simulink model "cosmic_ray_system_top"  (R2019a)
settings: Solver=VariableStepAuto  StartTime=0.0  StopTime=10.0  RelTol=1e-3
libraries: xbsIndex_r4 x3434, casper_library_misc x148, xps_library x3, casper_library_delays x1
(part 10 of 27)

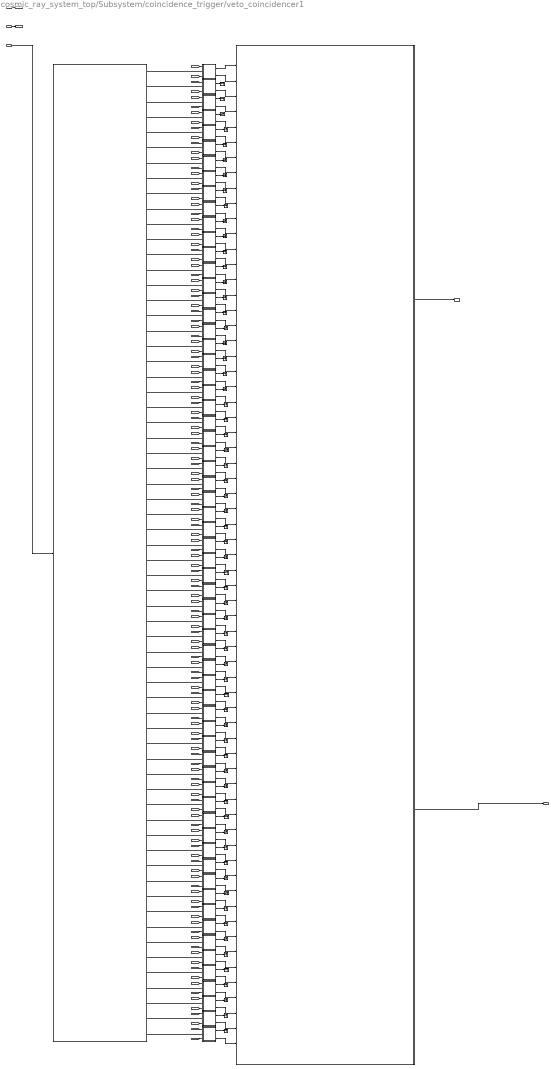
== system cosmic_ray_system_top/Subsystem/coincidence_trigger/veto_coincidencer1 ==
  window_length : Inport
  data_bus_in : Inport  Port=2
  sync_in : Inport  Port=3
  Terminator{,1..62} (63 alike) : Terminator
  adder_tree : Subsystem  AncestorBlock=casper_library_misc/adder_tree  mask(adder_tree){n_inputs=64, csp_latency=1, adder_imp=Fabric, first_stage_hdl=on, floating_point=off, dvalid_en=off, float_type=single, frac_width=0, exp_width=0}
      mask prompts: n_inputs "Number of Inputs"; csp_latency "Add Latency"; adder_imp "Adder implementation"; first_stage_hdl "Use behavioural HDL for first stage of adders"; floating_point "floating point"; float_type "float type"; frac_width "fraction length"; exp_width "exponent length"
      mask help:
      | Sums all inputs using a tree of adds and delays.
      |
      | Number of inputs: The number of inputs to the block to be summed
      | Add latency: The number of clock cycles to perform one addition (affects timing)..
      | Adder implementation: choice of fabric or DSP48E core, or behavioral HDL
      | Use behavioural HDL for first stage of adders: Causes the first stage of adders to be absorbed into DSP blocks if multipliers precede them (Virtex 5). Overrides Adder implementation
      mask init: same as cosmic_ray_system_top/Subsystem/coincidence_trigger/veto_coincidencer/adder_tree
      settings: AttributesFormatString=latency 6
      mask Help: eval('xlWeb(''http://casper.berkeley.edu/wiki/Adder_tree'')')
      mask TypeOptions adder_imp: Behavioral | Fabric | DSP48
      mask Callback floating_point:
      | onoff = get_param(gcb, 'floating_point');
      | if strcmp(onoff,'on')
      |     enable_fixpt = 'off'
      |     set_param_state(gcb, 'float_type', 'on')
      | 
      |     f_type = get_param(gcb, 'float_type')
      |     if strcmp(f_type,'custom')
      |         set_param_state(gcb, 'exp_width', 'on')
      |         set_param_state(gcb, 'frac_width', 'on')
      |     else
      |         set_param_state(gcb, 'exp_width', 'off')
      |         set_param_state(gcb, 'frac_width', 'off')
      |     end
      | 
      | 
      | else
      |     enable_fixpt = 'on'
      |     set_param_state(gcb, 'float_type', 'off')
      |     set_param_state(gcb, 'exp_width', 'off')
      |     set_param_state(gcb, 'frac_width', 'off')
      | end
      mask TypeOptions float_type: single | custom
      mask Callback float_type:
      | f_type = get_param(gcb, 'float_type')
      | if strcmp(f_type,'custom')
      |     set_param_state(gcb, 'exp_width', 'on')
      |     set_param_state(gcb, 'frac_width', 'on')
      | else
      |     set_param_state(gcb, 'exp_width', 'off')
      |     set_param_state(gcb, 'frac_width', 'off')
      | end
  bus_expand : Subsystem  AncestorBlock=casper_library_flow_control/bus_expand  mask(bus_expand){mode=divisions of equal size, outputNum=64, outputWidth=1, outputBinaryPt=0, outputArithmeticType=0, show_format=off, outputToWorkspace=off, variablePrefix=out, outputToModelAsWell=on}
      mask prompts: outputNum "Number of outputs:"; outputWidth "Output width:"; outputBinaryPt "Output binary point position:"; outputArithmeticType "Output arithmetic type (ufix=0, fix=1, bool=2):"; show_format "Print format string?"; outputToWorkspace "Output to workspace?"; variablePrefix "Variable name prefix:"; outputToModelAsWell "Output to model as well?"
      mask help:
      | Expands a 'bus' made using a bus_create or Xilinx
      | concat block.
      | The input will be divided into the specified number
      | of outputs with the specified arithmetic types.
      | Divisions are made from most significant bit.
      mask init: same as cosmic_ray_system_top/Subsystem/buffer_and_packetizer/bus_expand
      settings: AttributesFormatString=64 outputs
      mask TypeOptions mode: divisions of equal size | divisions of arbitrary size
      mask Callback mode: bus_expand_callback();
      mask Callback outputWidth: bus_expand_callback();
      mask Callback outputToWorkspace: bus_expand_callback();
  custom_pulse_extend_with_sync1 : Subsystem
  custom_pulse_extend_with_sync10 : Subsystem
  custom_pulse_extend_with_sync11 : Subsystem
  custom_pulse_extend_with_sync12 : Subsystem
  custom_pulse_extend_with_sync13 : Subsystem
  custom_pulse_extend_with_sync14 : Subsystem
  custom_pulse_extend_with_sync15 : Subsystem
  custom_pulse_extend_with_sync16 : Subsystem
  custom_pulse_extend_with_sync17 : Subsystem
  custom_pulse_extend_with_sync18 : Subsystem
  custom_pulse_extend_with_sync19 : Subsystem
  custom_pulse_extend_with_sync2 : Subsystem
  custom_pulse_extend_with_sync20 : Subsystem
  custom_pulse_extend_with_sync21 : Subsystem
  custom_pulse_extend_with_sync22 : Subsystem
  custom_pulse_extend_with_sync23 : Subsystem
  custom_pulse_extend_with_sync24 : Subsystem
  custom_pulse_extend_with_sync25 : Subsystem
  custom_pulse_extend_with_sync26 : Subsystem
  custom_pulse_extend_with_sync27 : Subsystem
  custom_pulse_extend_with_sync28 : Subsystem
  custom_pulse_extend_with_sync29 : Subsystem
  custom_pulse_extend_with_sync3 : Subsystem
  custom_pulse_extend_with_sync30 : Subsystem
  custom_pulse_extend_with_sync31 : Subsystem
  custom_pulse_extend_with_sync32 : Subsystem
  custom_pulse_extend_with_sync33 : Subsystem
  custom_pulse_extend_with_sync34 : Subsystem
  custom_pulse_extend_with_sync35 : Subsystem
  custom_pulse_extend_with_sync36 : Subsystem
  custom_pulse_extend_with_sync37 : Subsystem
  custom_pulse_extend_with_sync38 : Subsystem
  custom_pulse_extend_with_sync39 : Subsystem
  custom_pulse_extend_with_sync4 : Subsystem
  custom_pulse_extend_with_sync40 : Subsystem
  custom_pulse_extend_with_sync41 : Subsystem
  custom_pulse_extend_with_sync42 : Subsystem
  custom_pulse_extend_with_sync43 : Subsystem
  custom_pulse_extend_with_sync44 : Subsystem
  custom_pulse_extend_with_sync45 : Subsystem
  custom_pulse_extend_with_sync46 : Subsystem
  custom_pulse_extend_with_sync47 : Subsystem
  custom_pulse_extend_with_sync48 : Subsystem
  custom_pulse_extend_with_sync49 : Subsystem
  custom_pulse_extend_with_sync5 : Subsystem
  custom_pulse_extend_with_sync50 : Subsystem
  custom_pulse_extend_with_sync51 : Subsystem
  custom_pulse_extend_with_sync52 : Subsystem
  custom_pulse_extend_with_sync53 : Subsystem
  custom_pulse_extend_with_sync54 : Subsystem
  custom_pulse_extend_with_sync55 : Subsystem
  custom_pulse_extend_with_sync56 : Subsystem
  custom_pulse_extend_with_sync57 : Subsystem
  custom_pulse_extend_with_sync58 : Subsystem
  custom_pulse_extend_with_sync59 : Subsystem
  custom_pulse_extend_with_sync6 : Subsystem
  custom_pulse_extend_with_sync60 : Subsystem
  custom_pulse_extend_with_sync61 : Subsystem
  custom_pulse_extend_with_sync62 : Subsystem
  custom_pulse_extend_with_sync63 : Subsystem
  custom_pulse_extend_with_sync64 : Subsystem
  custom_pulse_extend_with_sync7 : Subsystem
  custom_pulse_extend_with_sync8 : Subsystem
  custom_pulse_extend_with_sync9 : Subsystem
  sync_out : Outport
  "out " : Outport  Port=2
  wires:
  custom_pulse_extend_with_sync63/2("out ") -> adder_tree/65(din64)
  custom_pulse_extend_with_sync64/2("out ") -> adder_tree/64(din63)
  custom_pulse_extend_with_sync61/2("out ") -> adder_tree/63(din62)
  custom_pulse_extend_with_sync62/2("out ") -> adder_tree/62(din61)
  custom_pulse_extend_with_sync44/2("out ") -> adder_tree/61(din60)
  custom_pulse_extend_with_sync45/2("out ") -> adder_tree/60(din59)
  custom_pulse_extend_with_sync41/2("out ") -> adder_tree/59(din58)
  custom_pulse_extend_with_sync43/2("out ") -> adder_tree/58(din57)
  custom_pulse_extend_with_sync39/2("out ") -> adder_tree/57(din56)
  custom_pulse_extend_with_sync40/2("out ") -> adder_tree/56(din55)
  custom_pulse_extend_with_sync54/2("out ") -> adder_tree/55(din54)
  custom_pulse_extend_with_sync51/2("out ") -> adder_tree/54(din53)
  custom_pulse_extend_with_sync52/2("out ") -> adder_tree/53(din52)
  custom_pulse_extend_with_sync49/2("out ") -> adder_tree/52(din51)
  custom_pulse_extend_with_sync50/2("out ") -> adder_tree/51(din50)
  custom_pulse_extend_with_sync47/2("out ") -> adder_tree/50(din49)
  custom_pulse_extend_with_sync48/2("out ") -> adder_tree/49(din48)
  custom_pulse_extend_with_sync38/2("out ") -> adder_tree/48(din47)
  custom_pulse_extend_with_sync46/2("out ") -> adder_tree/47(din46)
  custom_pulse_extend_with_sync36/2("out ") -> adder_tree/46(din45)
  custom_pulse_extend_with_sync37/2("out ") -> adder_tree/45(din44)
  custom_pulse_extend_with_sync34/2("out ") -> adder_tree/44(din43)
  custom_pulse_extend_with_sync35/2("out ") -> adder_tree/43(din42)
  custom_pulse_extend_with_sync32/2("out ") -> adder_tree/42(din41)
  custom_pulse_extend_with_sync33/2("out ") -> adder_tree/41(din40)
  custom_pulse_extend_with_sync60/2("out ") -> adder_tree/40(din39)
  custom_pulse_extend_with_sync58/2("out ") -> adder_tree/39(din38)
  custom_pulse_extend_with_sync59/2("out ") -> adder_tree/38(din37)
  custom_pulse_extend_with_sync56/2("out ") -> adder_tree/37(din36)
  custom_pulse_extend_with_sync57/2("out ") -> adder_tree/36(din35)
  custom_pulse_extend_with_sync53/2("out ") -> adder_tree/35(din34)
  custom_pulse_extend_with_sync55/2("out ") -> adder_tree/34(din33)
  custom_pulse_extend_with_sync31/2("out ") -> adder_tree/33(din32)
  custom_pulse_extend_with_sync42/2("out ") -> adder_tree/32(din31)
  custom_pulse_extend_with_sync21/2("out ") -> adder_tree/31(din30)
  custom_pulse_extend_with_sync22/2("out ") -> adder_tree/30(din29)
  custom_pulse_extend_with_sync19/2("out ") -> adder_tree/29(din28)
  custom_pulse_extend_with_sync20/2("out ") -> adder_tree/28(din27)
  custom_pulse_extend_with_sync17/2("out ") -> adder_tree/27(din26)
  custom_pulse_extend_with_sync18/2("out ") -> adder_tree/26(din25)
  custom_pulse_extend_with_sync30/2("out ") -> adder_tree/25(din24)
  custom_pulse_extend_with_sync28/2("out ") -> adder_tree/24(din23)
  custom_pulse_extend_with_sync29/2("out ") -> adder_tree/23(din22)
  custom_pulse_extend_with_sync26/2("out ") -> adder_tree/22(din21)
  custom_pulse_extend_with_sync27/2("out ") -> adder_tree/21(din20)
  custom_pulse_extend_with_sync24/2("out ") -> adder_tree/20(din19)
  custom_pulse_extend_with_sync25/2("out ") -> adder_tree/19(din18)
  custom_pulse_extend_with_sync16/2("out ") -> adder_tree/18(din17)
  custom_pulse_extend_with_sync23/2("out ") -> adder_tree/17(din16)
  custom_pulse_extend_with_sync14/2("out ") -> adder_tree/16(din15)
  custom_pulse_extend_with_sync15/2("out ") -> adder_tree/15(din14)
  custom_pulse_extend_with_sync12/2("out ") -> adder_tree/14(din13)
  custom_pulse_extend_with_sync13/2("out ") -> adder_tree/13(din12)
  custom_pulse_extend_with_sync10/2("out ") -> adder_tree/12(din11)
  custom_pulse_extend_with_sync11/2("out ") -> adder_tree/11(din10)
  custom_pulse_extend_with_sync9/2("out ") -> adder_tree/10(din9)
  custom_pulse_extend_with_sync7/2("out ") -> adder_tree/9(din8)
  custom_pulse_extend_with_sync8/2("out ") -> adder_tree/8(din7)
  custom_pulse_extend_with_sync5/2("out ") -> adder_tree/7(din6)
  custom_pulse_extend_with_sync6/2("out ") -> adder_tree/6(din5)
  custom_pulse_extend_with_sync3/2("out ") -> adder_tree/5(din4)
  custom_pulse_extend_with_sync4/2("out ") -> adder_tree/4(din3)
  custom_pulse_extend_with_sync1/2("out ") -> adder_tree/3(din2)
  custom_pulse_extend_with_sync2/2("out ") -> adder_tree/2(din1)
  custom_pulse_extend_with_sync44/1(sync_out) -> Terminator61/1
  custom_pulse_extend_with_sync62/1(sync_out) -> Terminator62/1
  custom_pulse_extend_with_sync61/1(sync_out) -> Terminator58/1
  custom_pulse_extend_with_sync64/1(sync_out) -> Terminator59/1
  custom_pulse_extend_with_sync63/1(sync_out) -> Terminator60/1
  custom_pulse_extend_with_sync45/1(sync_out) -> Terminator55/1
  custom_pulse_extend_with_sync41/1(sync_out) -> Terminator54/1
  custom_pulse_extend_with_sync43/1(sync_out) -> Terminator53/1
  custom_pulse_extend_with_sync39/1(sync_out) -> Terminator57/1
  custom_pulse_extend_with_sync40/1(sync_out) -> Terminator56/1
  custom_pulse_extend_with_sync60/1(sync_out) -> Terminator40/1
  custom_pulse_extend_with_sync33/1(sync_out) -> Terminator41/1
  custom_pulse_extend_with_sync32/1(sync_out) -> Terminator42/1
  custom_pulse_extend_with_sync46/1(sync_out) -> Terminator39/1
  custom_pulse_extend_with_sync36/1(sync_out) -> Terminator38/1
  custom_pulse_extend_with_sync37/1(sync_out) -> Terminator37/1
  custom_pulse_extend_with_sync34/1(sync_out) -> Terminator44/1
  custom_pulse_extend_with_sync35/1(sync_out) -> Terminator43/1
  custom_pulse_extend_with_sync50/1(sync_out) -> Terminator51/1
  custom_pulse_extend_with_sync49/1(sync_out) -> Terminator52/1
  custom_pulse_extend_with_sync52/1(sync_out) -> Terminator45/1
  custom_pulse_extend_with_sync51/1(sync_out) -> Terminator46/1
  custom_pulse_extend_with_sync54/1(sync_out) -> Terminator47/1
  custom_pulse_extend_with_sync47/1(sync_out) -> Terminator50/1
  custom_pulse_extend_with_sync48/1(sync_out) -> Terminator49/1
  custom_pulse_extend_with_sync38/1(sync_out) -> Terminator48/1
  custom_pulse_extend_with_sync42/1(sync_out) -> Terminator32/1
  custom_pulse_extend_with_sync31/1(sync_out) -> Terminator33/1
  custom_pulse_extend_with_sync55/1(sync_out) -> Terminator34/1
  custom_pulse_extend_with_sync58/1(sync_out) -> Terminator31/1
  custom_pulse_extend_with_sync59/1(sync_out) -> Terminator30/1
  custom_pulse_extend_with_sync56/1(sync_out) -> Terminator29/1
  custom_pulse_extend_with_sync57/1(sync_out) -> Terminator36/1
  custom_pulse_extend_with_sync53/1(sync_out) -> Terminator35/1
  custom_pulse_extend_with_sync17/1(sync_out) -> Terminator27/1
  custom_pulse_extend_with_sync20/1(sync_out) -> Terminator28/1
  custom_pulse_extend_with_sync19/1(sync_out) -> Terminator21/1
  custom_pulse_extend_with_sync22/1(sync_out) -> Terminator22/1
  custom_pulse_extend_with_sync21/1(sync_out) -> Terminator23/1
  custom_pulse_extend_with_sync18/1(sync_out) -> Terminator26/1
  custom_pulse_extend_with_sync30/1(sync_out) -> Terminator25/1
  custom_pulse_extend_with_sync28/1(sync_out) -> Terminator24/1
  custom_pulse_extend_with_sync14/1(sync_out) -> Terminator16/1
  custom_pulse_extend_with_sync23/1(sync_out) -> Terminator17/1
  custom_pulse_extend_with_sync16/1(sync_out) -> Terminator18/1
  custom_pulse_extend_with_sync29/1(sync_out) -> Terminator15/1
  custom_pulse_extend_with_sync26/1(sync_out) -> Terminator14/1
  custom_pulse_extend_with_sync27/1(sync_out) -> Terminator13/1
  custom_pulse_extend_with_sync24/1(sync_out) -> Terminator20/1
  custom_pulse_extend_with_sync25/1(sync_out) -> Terminator19/1
  custom_pulse_extend_with_sync11/1(sync_out) -> Terminator8/1
  custom_pulse_extend_with_sync10/1(sync_out) -> Terminator9/1
  custom_pulse_extend_with_sync13/1(sync_out) -> Terminator10/1
  custom_pulse_extend_with_sync12/1(sync_out) -> Terminator11/1
  custom_pulse_extend_with_sync15/1(sync_out) -> Terminator12/1
  custom_pulse_extend_with_sync9/1(sync_out) -> Terminator7/1
  custom_pulse_extend_with_sync7/1(sync_out) -> Terminator6/1
  custom_pulse_extend_with_sync8/1(sync_out) -> Terminator5/1
  custom_pulse_extend_with_sync5/1(sync_out) -> Terminator4/1
  custom_pulse_extend_with_sync6/1(sync_out) -> Terminator3/1
  custom_pulse_extend_with_sync3/1(sync_out) -> Terminator2/1
  custom_pulse_extend_with_sync4/1(sync_out) -> Terminator1/1
  custom_pulse_extend_with_sync1/1(sync_out) -> Terminator/1
  bus_expand/61(out4) -> custom_pulse_extend_with_sync62/2("in ")
  [sync] -> custom_pulse_extend_with_sync62/1(sync_in)
  [len] -> custom_pulse_extend_with_sync62/3("pulse_length ")
  [len] -> custom_pulse_extend_with_sync61/3("pulse_length ")
  [sync] -> custom_pulse_extend_with_sync61/1(sync_in)
  bus_expand/62(out3) -> custom_pulse_extend_with_sync61/2("in ")
  bus_expand/64(lsb_out1) -> custom_pulse_extend_with_sync63/2("in ")
  [sync] -> custom_pulse_extend_with_sync63/1(sync_in)
  [len] -> custom_pulse_extend_with_sync63/3("pulse_length ")
  [len] -> custom_pulse_extend_with_sync64/3("pulse_length ")
  [sync] -> custom_pulse_extend_with_sync64/1(sync_in)
  bus_expand/63(out2) -> custom_pulse_extend_with_sync64/2("in ")
  bus_expand/31(out34) -> custom_pulse_extend_with_sync42/2("in ")
  [sync] -> custom_pulse_extend_with_sync42/1(sync_in)
  [len] -> custom_pulse_extend_with_sync42/3("pulse_length ")
  [len] -> custom_pulse_extend_with_sync31/3("pulse_length ")
  [sync] -> custom_pulse_extend_with_sync31/1(sync_in)
  bus_expand/32(out33) -> custom_pulse_extend_with_sync31/2("in ")
  bus_expand/34(out31) -> custom_pulse_extend_with_sync53/2("in ")
  [sync] -> custom_pulse_extend_with_sync53/1(sync_in)
  [len] -> custom_pulse_extend_with_sync53/3("pulse_length ")
  [len] -> custom_pulse_extend_with_sync55/3("pulse_length ")
  [sync] -> custom_pulse_extend_with_sync55/1(sync_in)
  bus_expand/33(out32) -> custom_pulse_extend_with_sync55/2("in ")
  bus_expand/37(out28) -> custom_pulse_extend_with_sync59/2("in ")
  [sync] -> custom_pulse_extend_with_sync59/1(sync_in)
  [len] -> custom_pulse_extend_with_sync59/3("pulse_length ")
  [len] -> custom_pulse_extend_with_sync58/3("pulse_length ")
  [sync] -> custom_pulse_extend_with_sync58/1(sync_in)
  bus_expand/38(out27) -> custom_pulse_extend_with_sync58/2("in ")
  bus_expand/36(out29) -> custom_pulse_extend_with_sync56/2("in ")
  [sync] -> custom_pulse_extend_with_sync56/1(sync_in)
  [len] -> custom_pulse_extend_with_sync56/3("pulse_length ")
  [len] -> custom_pulse_extend_with_sync57/3("pulse_length ")
  [sync] -> custom_pulse_extend_with_sync57/1(sync_in)
  bus_expand/35(out30) -> custom_pulse_extend_with_sync57/2("in ")
  bus_expand/42(out23) -> custom_pulse_extend_with_sync35/2("in ")
  [sync] -> custom_pulse_extend_with_sync35/1(sync_in)
  [len] -> custom_pulse_extend_with_sync35/3("pulse_length ")
  [len] -> custom_pulse_extend_with_sync34/3("pulse_length ")
  [sync] -> custom_pulse_extend_with_sync34/1(sync_in)
  bus_expand/43(out22) -> custom_pulse_extend_with_sync34/2("in ")
  bus_expand/45(out20) -> custom_pulse_extend_with_sync36/2("in ")
  [sync] -> custom_pulse_extend_with_sync36/1(sync_in)
  [len] -> custom_pulse_extend_with_sync36/3("pulse_length ")
  [len] -> custom_pulse_extend_with_sync37/3("pulse_length ")
  [sync] -> custom_pulse_extend_with_sync37/1(sync_in)
  bus_expand/44(out21) -> custom_pulse_extend_with_sync37/2("in ")
  bus_expand/40(out25) -> custom_pulse_extend_with_sync33/2("in ")
  [sync] -> custom_pulse_extend_with_sync33/1(sync_in)
  [len] -> custom_pulse_extend_with_sync33/3("pulse_length ")
  [len] -> custom_pulse_extend_with_sync32/3("pulse_length ")
  [sync] -> custom_pulse_extend_with_sync32/1(sync_in)
  bus_expand/41(out24) -> custom_pulse_extend_with_sync32/2("in ")
  bus_expand/39(out26) -> custom_pulse_extend_with_sync60/2("in ")
  [sync] -> custom_pulse_extend_with_sync60/1(sync_in)
  [len] -> custom_pulse_extend_with_sync60/3("pulse_length ")
  [len] -> custom_pulse_extend_with_sync54/3("pulse_length ")
  [sync] -> custom_pulse_extend_with_sync54/1(sync_in)
  bus_expand/54(out11) -> custom_pulse_extend_with_sync54/2("in ")
  bus_expand/56(out9) -> custom_pulse_extend_with_sync39/2("in ")
  [sync] -> custom_pulse_extend_with_sync39/1(sync_in)
  [len] -> custom_pulse_extend_with_sync39/3("pulse_length ")
  [len] -> custom_pulse_extend_with_sync40/3("pulse_length ")
  [sync] -> custom_pulse_extend_with_sync40/1(sync_in)
  bus_expand/55(out10) -> custom_pulse_extend_with_sync40/2("in ")
  bus_expand/59(out6) -> custom_pulse_extend_with_sync45/2("in ")
  [sync] -> custom_pulse_extend_with_sync45/1(sync_in)
  [len] -> custom_pulse_extend_with_sync45/3("pulse_length ")
  [len] -> custom_pulse_extend_with_sync44/3("pulse_length ")
  [sync] -> custom_pulse_extend_with_sync44/1(sync_in)
  bus_expand/60(out5) -> custom_pulse_extend_with_sync44/2("in ")
  bus_expand/58(out7) -> custom_pulse_extend_with_sync41/2("in ")
  [sync] -> custom_pulse_extend_with_sync41/1(sync_in)
  [len] -> custom_pulse_extend_with_sync41/3("pulse_length ")
  [len] -> custom_pulse_extend_with_sync43/3("pulse_length ")
  [sync] -> custom_pulse_extend_with_sync43/1(sync_in)
  bus_expand/57(out8) -> custom_pulse_extend_with_sync43/2("in ")
  bus_expand/50(out15) -> custom_pulse_extend_with_sync50/2("in ")
  [sync] -> custom_pulse_extend_with_sync50/1(sync_in)
  [len] -> custom_pulse_extend_with_sync50/3("pulse_length ")
  [len] -> custom_pulse_extend_with_sync49/3("pulse_length ")
  [sync] -> custom_pulse_extend_with_sync49/1(sync_in)
  bus_expand/51(out14) -> custom_pulse_extend_with_sync49/2("in ")
  bus_expand/53(out12) -> custom_pulse_extend_with_sync51/2("in ")
  [sync] -> custom_pulse_extend_with_sync51/1(sync_in)
  [len] -> custom_pulse_extend_with_sync51/3("pulse_length ")
  [len] -> custom_pulse_extend_with_sync52/3("pulse_length ")
  [sync] -> custom_pulse_extend_with_sync52/1(sync_in)
  bus_expand/52(out13) -> custom_pulse_extend_with_sync52/2("in ")
  bus_expand/48(out17) -> custom_pulse_extend_with_sync48/2("in ")
  [sync] -> custom_pulse_extend_with_sync48/1(sync_in)
  [len] -> custom_pulse_extend_with_sync48/3("pulse_length ")
  [len] -> custom_pulse_extend_with_sync47/3("pulse_length ")
  [sync] -> custom_pulse_extend_with_sync47/1(sync_in)
  bus_expand/49(out16) -> custom_pulse_extend_with_sync47/2("in ")
  bus_expand/47(out18) -> custom_pulse_extend_with_sync38/2("in ")
  [sync] -> custom_pulse_extend_with_sync38/1(sync_in)
  [len] -> custom_pulse_extend_with_sync38/3("pulse_length ")
  [len] -> custom_pulse_extend_with_sync46/3("pulse_length ")
  [sync] -> custom_pulse_extend_with_sync46/1(sync_in)
  bus_expand/46(out19) -> custom_pulse_extend_with_sync46/2("in ")
  bus_expand/16(out49) -> custom_pulse_extend_with_sync23/2("in ")
  [sync] -> custom_pulse_extend_with_sync23/1(sync_in)
  [len] -> custom_pulse_extend_with_sync23/3("pulse_length ")
  [len] -> custom_pulse_extend_with_sync16/3("pulse_length ")
  [sync] -> custom_pulse_extend_with_sync16/1(sync_in)
  bus_expand/17(out48) -> custom_pulse_extend_with_sync16/2("in ")
  bus_expand/19(out46) -> custom_pulse_extend_with_sync24/2("in ")
  [sync] -> custom_pulse_extend_with_sync24/1(sync_in)
  [len] -> custom_pulse_extend_with_sync24/3("pulse_length ")
  [len] -> custom_pulse_extend_with_sync25/3("pulse_length ")
  [sync] -> custom_pulse_extend_with_sync25/1(sync_in)
  bus_expand/18(out47) -> custom_pulse_extend_with_sync25/2("in ")
  bus_expand/22(out43) -> custom_pulse_extend_with_sync29/2("in ")
  [sync] -> custom_pulse_extend_with_sync29/1(sync_in)
  [len] -> custom_pulse_extend_with_sync29/3("pulse_length ")
  [len] -> custom_pulse_extend_with_sync28/3("pulse_length ")
  [sync] -> custom_pulse_extend_with_sync28/1(sync_in)
  bus_expand/23(out42) -> custom_pulse_extend_with_sync28/2("in ")
  bus_expand/21(out44) -> custom_pulse_extend_with_sync26/2("in ")
  [sync] -> custom_pulse_extend_with_sync26/1(sync_in)
  [len] -> custom_pulse_extend_with_sync26/3("pulse_length ")
  [len] -> custom_pulse_extend_with_sync27/3("pulse_length ")
  [sync] -> custom_pulse_extend_with_sync27/1(sync_in)
  bus_expand/20(out45) -> custom_pulse_extend_with_sync27/2("in ")
  bus_expand/27(out38) -> custom_pulse_extend_with_sync20/2("in ")
  [sync] -> custom_pulse_extend_with_sync20/1(sync_in)
  [len] -> custom_pulse_extend_with_sync20/3("pulse_length ")
  [len] -> custom_pulse_extend_with_sync19/3("pulse_length ")
  [sync] -> custom_pulse_extend_with_sync19/1(sync_in)
  bus_expand/28(out37) -> custom_pulse_extend_with_sync19/2("in ")
  bus_expand/30(out35) -> custom_pulse_extend_with_sync21/2("in ")
  [sync] -> custom_pulse_extend_with_sync21/1(sync_in)
  [len] -> custom_pulse_extend_with_sync21/3("pulse_length ")
  [len] -> custom_pulse_extend_with_sync22/3("pulse_length ")
  [sync] -> custom_pulse_extend_with_sync22/1(sync_in)
  bus_expand/29(out36) -> custom_pulse_extend_with_sync22/2("in ")
  bus_expand/25(out40) -> custom_pulse_extend_with_sync18/2("in ")
  [sync] -> custom_pulse_extend_with_sync18/1(sync_in)
  [len] -> custom_pulse_extend_with_sync18/3("pulse_length ")
  [len] -> custom_pulse_extend_with_sync17/3("pulse_length ")
  [sync] -> custom_pulse_extend_with_sync17/1(sync_in)
  bus_expand/26(out39) -> custom_pulse_extend_with_sync17/2("in ")
  bus_expand/24(out41) -> custom_pulse_extend_with_sync30/2("in ")
  [sync] -> custom_pulse_extend_with_sync30/1(sync_in)
  [len] -> custom_pulse_extend_with_sync30/3("pulse_length ")
  [len] -> custom_pulse_extend_with_sync9/3("pulse_length ")
  [sync] -> custom_pulse_extend_with_sync9/1(sync_in)
  bus_expand/9(out56) -> custom_pulse_extend_with_sync9/2("in ")
  bus_expand/11(out54) -> custom_pulse_extend_with_sync10/2("in ")
  [sync] -> custom_pulse_extend_with_sync10/1(sync_in)
  [len] -> custom_pulse_extend_with_sync10/3("pulse_length ")
  [len] -> custom_pulse_extend_with_sync11/3("pulse_length ")
  [sync] -> custom_pulse_extend_with_sync11/1(sync_in)
  bus_expand/10(out55) -> custom_pulse_extend_with_sync11/2("in ")
  bus_expand/14(out51) -> custom_pulse_extend_with_sync15/2("in ")
  [sync] -> custom_pulse_extend_with_sync15/1(sync_in)
  [len] -> custom_pulse_extend_with_sync15/3("pulse_length ")
  [len] -> custom_pulse_extend_with_sync14/3("pulse_length ")
  [sync] -> custom_pulse_extend_with_sync14/1(sync_in)
  bus_expand/15(out50) -> custom_pulse_extend_with_sync14/2("in ")
  bus_expand/13(out52) -> custom_pulse_extend_with_sync12/2("in ")
  [sync] -> custom_pulse_extend_with_sync12/1(sync_in)
  [len] -> custom_pulse_extend_with_sync12/3("pulse_length ")
  [len] -> custom_pulse_extend_with_sync13/3("pulse_length ")
  [sync] -> custom_pulse_extend_with_sync13/1(sync_in)
  bus_expand/12(out53) -> custom_pulse_extend_with_sync13/2("in ")
  bus_expand/5(out60) -> custom_pulse_extend_with_sync6/2("in ")
  [sync] -> custom_pulse_extend_with_sync6/1(sync_in)
  [len] -> custom_pulse_extend_with_sync6/3("pulse_length ")
  [len] -> custom_pulse_extend_with_sync5/3("pulse_length ")
  [sync] -> custom_pulse_extend_with_sync5/1(sync_in)
  bus_expand/6(out59) -> custom_pulse_extend_with_sync5/2("in ")
  bus_expand/8(out57) -> custom_pulse_extend_with_sync7/2("in ")
  [sync] -> custom_pulse_extend_with_sync7/1(sync_in)
  [len] -> custom_pulse_extend_with_sync7/3("pulse_length ")
  [len] -> custom_pulse_extend_with_sync8/3("pulse_length ")
  [sync] -> custom_pulse_extend_with_sync8/1(sync_in)
  bus_expand/7(out58) -> custom_pulse_extend_with_sync8/2("in ")
  bus_expand/3(out62) -> custom_pulse_extend_with_sync4/2("in ")
  [sync] -> custom_pulse_extend_with_sync4/1(sync_in)
  [len] -> custom_pulse_extend_with_sync4/3("pulse_length ")
  [len] -> custom_pulse_extend_with_sync3/3("pulse_length ")
  [sync] -> custom_pulse_extend_with_sync3/1(sync_in)
  bus_expand/4(out61) -> custom_pulse_extend_with_sync3/2("in ")
  bus_expand/2(out63) -> custom_pulse_extend_with_sync1/2("in ")
  [sync] -> custom_pulse_extend_with_sync1/1(sync_in)
  [len] -> custom_pulse_extend_with_sync1/3("pulse_length ")
  [len] -> custom_pulse_extend_with_sync2/3("pulse_length ")
  [sync] -> custom_pulse_extend_with_sync2/1(sync_in)
  sync_in/1 -> [sync]
  window_length/1 -> [len]
  bus_expand/1(msb_out64) -> custom_pulse_extend_with_sync2/2("in ")
  data_bus_in/1 -> bus_expand/1(bus_in)
  adder_tree/2(dout) -> "out "/1
  adder_tree/1(sync_out) -> sync_out/1
  custom_pulse_extend_with_sync2/1(sync_out) -> adder_tree/1(sync)

== system cosmic_ray_system_top/Subsystem/constant_test_signal1/bus_create ==
  in1 : Inport
  in2 : Inport  Port=2
  in3 : Inport  Port=3
  in4 : Inport  Port=4
  in5 : Inport  Port=5
  in6 : Inport  Port=6
  in7 : Inport  Port=7
  in8 : Inport  Port=8
  in9 : Inport  Port=9
  in10 : Inport  Port=10
  in11 : Inport  Port=11
  in12 : Inport  Port=12
  in13 : Inport  Port=13
  in14 : Inport  Port=14
  in15 : Inport  Port=15
  in16 : Inport  Port=16
  in17 : Inport  Port=17
  in18 : Inport  Port=18
  in19 : Inport  Port=19
  in20 : Inport  Port=20
  in21 : Inport  Port=21
  in22 : Inport  Port=22
  in23 : Inport  Port=23
  in24 : Inport  Port=24
  in25 : Inport  Port=25
  in26 : Inport  Port=26
  in27 : Inport  Port=27
  in28 : Inport  Port=28
  in29 : Inport  Port=29
  in30 : Inport  Port=30
  in31 : Inport  Port=31
  in32 : Inport  Port=32
  in33 : Inport  Port=33
  in34 : Inport  Port=34
  in35 : Inport  Port=35
  in36 : Inport  Port=36
  in37 : Inport  Port=37
  in38 : Inport  Port=38
  in39 : Inport  Port=39
  in40 : Inport  Port=40
  in41 : Inport  Port=41
  in42 : Inport  Port=42
  in43 : Inport  Port=43
  in44 : Inport  Port=44
  in45 : Inport  Port=45
  in46 : Inport  Port=46
  in47 : Inport  Port=47
  in48 : Inport  Port=48
  in49 : Inport  Port=49
  in50 : Inport  Port=50
  in51 : Inport  Port=51
  in52 : Inport  Port=52
  in53 : Inport  Port=53
  in54 : Inport  Port=54
  in55 : Inport  Port=55
  in56 : Inport  Port=56
  in57 : Inport  Port=57
  in58 : Inport  Port=58
  in59 : Inport  Port=59
  in60 : Inport  Port=60
  in61 : Inport  Port=61
  in62 : Inport  Port=62
  in63 : Inport  Port=63
  in64 : Inport  Port=64
  concatenate : xbsIndex_r4/Concat  num_inputs=64  dbl_ovrd=off  block_type=concat
  reinterpret{1..64} (64 alike) : xbsIndex_r4/Reinterpret  force_arith_type=on  arith_type=Unsigned  force_bin_pt=on  bin_pt=0  block_type=reinterpret
      reinterpret1 settings: infoedit="Changes signal type without altering the binary representation.   You can changed the signal between signed and unsigned, and relocate the binary point.<br><br>Hardware notes: In hardware this block costs nothing.<br><br>Example:  Suppose the input is 6 bits wide, signed, with 2 fractional bits, and the output is forced to unsigned with 0 fractional bits.  Then an input of -2.0 (1110.00 in binary 2's complement) becomes an output of 56 (111000 in binary)."
      reinterpret2 settings: infoedit="Changes signal type without altering the binary representation.   You can changed the signal between signed and unsigned, and relocate the binary point.<br><br>Hardware notes: In hardware this block costs nothing.<br><br>Example:  Suppose the input is 6 bits wide, signed, with 2 fractional bits, and the output is forced to unsigned with 0 fractional bits.  Then an input of -2.0 (1110.00 in binary 2's complement) becomes an output of 56 (111000 in binary)."
  bus_out : Outport
  wires:
  concatenate/1 -> bus_out/1
  in1/1 -> reinterpret1/1
  reinterpret1/1 -> concatenate/1
  in2/1 -> reinterpret2/1
  reinterpret2/1 -> concatenate/2
  in3/1 -> reinterpret3/1
  reinterpret3/1 -> concatenate/3
  in4/1 -> reinterpret4/1
  reinterpret4/1 -> concatenate/4
  in5/1 -> reinterpret5/1
  reinterpret5/1 -> concatenate/5
  in6/1 -> reinterpret6/1
  reinterpret6/1 -> concatenate/6
  in7/1 -> reinterpret7/1
  reinterpret7/1 -> concatenate/7
  in8/1 -> reinterpret8/1
  reinterpret8/1 -> concatenate/8
  in9/1 -> reinterpret9/1
  reinterpret9/1 -> concatenate/9
  in10/1 -> reinterpret10/1
  reinterpret10/1 -> concatenate/10
  in11/1 -> reinterpret11/1
  reinterpret11/1 -> concatenate/11
  in12/1 -> reinterpret12/1
  reinterpret12/1 -> concatenate/12
  in13/1 -> reinterpret13/1
  reinterpret13/1 -> concatenate/13
  in14/1 -> reinterpret14/1
  reinterpret14/1 -> concatenate/14
  in15/1 -> reinterpret15/1
  reinterpret15/1 -> concatenate/15
  in16/1 -> reinterpret16/1
  reinterpret16/1 -> concatenate/16
  in17/1 -> reinterpret17/1
  reinterpret17/1 -> concatenate/17
  in18/1 -> reinterpret18/1
  reinterpret18/1 -> concatenate/18
  in19/1 -> reinterpret19/1
  reinterpret19/1 -> concatenate/19
  in20/1 -> reinterpret20/1
  reinterpret20/1 -> concatenate/20
  in21/1 -> reinterpret21/1
  reinterpret21/1 -> concatenate/21
  in22/1 -> reinterpret22/1
  reinterpret22/1 -> concatenate/22
  in23/1 -> reinterpret23/1
  reinterpret23/1 -> concatenate/23
  in24/1 -> reinterpret24/1
  reinterpret24/1 -> concatenate/24
  in25/1 -> reinterpret25/1
  reinterpret25/1 -> concatenate/25
  in26/1 -> reinterpret26/1
  reinterpret26/1 -> concatenate/26
  in27/1 -> reinterpret27/1
  reinterpret27/1 -> concatenate/27
  in28/1 -> reinterpret28/1
  reinterpret28/1 -> concatenate/28
  in29/1 -> reinterpret29/1
  reinterpret29/1 -> concatenate/29
  in30/1 -> reinterpret30/1
  reinterpret30/1 -> concatenate/30
  in31/1 -> reinterpret31/1
  reinterpret31/1 -> concatenate/31
  in32/1 -> reinterpret32/1
  reinterpret32/1 -> concatenate/32
  in33/1 -> reinterpret33/1
  reinterpret33/1 -> concatenate/33
  in34/1 -> reinterpret34/1
  reinterpret34/1 -> concatenate/34
  in35/1 -> reinterpret35/1
  reinterpret35/1 -> concatenate/35
  in36/1 -> reinterpret36/1
  reinterpret36/1 -> concatenate/36
  in37/1 -> reinterpret37/1
  reinterpret37/1 -> concatenate/37
  in38/1 -> reinterpret38/1
  reinterpret38/1 -> concatenate/38
  in39/1 -> reinterpret39/1
  reinterpret39/1 -> concatenate/39
  in40/1 -> reinterpret40/1
  reinterpret40/1 -> concatenate/40
  in41/1 -> reinterpret41/1
  reinterpret41/1 -> concatenate/41
  in42/1 -> reinterpret42/1
  reinterpret42/1 -> concatenate/42
  in43/1 -> reinterpret43/1
  reinterpret43/1 -> concatenate/43
  in44/1 -> reinterpret44/1
  reinterpret44/1 -> concatenate/44
  in45/1 -> reinterpret45/1
  reinterpret45/1 -> concatenate/45
  in46/1 -> reinterpret46/1
  reinterpret46/1 -> concatenate/46
  in47/1 -> reinterpret47/1
  reinterpret47/1 -> concatenate/47
  in48/1 -> reinterpret48/1
  reinterpret48/1 -> concatenate/48
  in49/1 -> reinterpret49/1
  reinterpret49/1 -> concatenate/49
  in50/1 -> reinterpret50/1
  reinterpret50/1 -> concatenate/50
  in51/1 -> reinterpret51/1
  reinterpret51/1 -> concatenate/51
  in52/1 -> reinterpret52/1
  reinterpret52/1 -> concatenate/52
  in53/1 -> reinterpret53/1
  reinterpret53/1 -> concatenate/53
  in54/1 -> reinterpret54/1
  reinterpret54/1 -> concatenate/54
  in55/1 -> reinterpret55/1
  reinterpret55/1 -> concatenate/55
  in56/1 -> reinterpret56/1
  reinterpret56/1 -> concatenate/56
  in57/1 -> reinterpret57/1
  reinterpret57/1 -> concatenate/57
  in58/1 -> reinterpret58/1
  reinterpret58/1 -> concatenate/58
  in59/1 -> reinterpret59/1
  reinterpret59/1 -> concatenate/59
  in60/1 -> reinterpret60/1
  reinterpret60/1 -> concatenate/60
  in61/1 -> reinterpret61/1
  reinterpret61/1 -> concatenate/61
  in62/1 -> reinterpret62/1
  reinterpret62/1 -> concatenate/62
  in63/1 -> reinterpret63/1
  reinterpret63/1 -> concatenate/63
  in64/1 -> reinterpret64/1
  reinterpret64/1 -> concatenate/64

== system cosmic_ray_system_top/Subsystem/core_trigger_timestamps/calc_add ==
  note: Use behavioural HDL
      | so that gets optimised
      | to minimum logic
  note: If reading/writing words
      | smaller than 32 bits,
      | change address so
      | that addressing is
      | big endian instead of
      | little, otherwise
      | pass through
  in : Inport
  add_sub : xbsIndex_r4/AddSub  mode=Subtraction  use_carryin=off  use_carryout=off  en=off  latency=0  precision=User Defined  arith_type=Unsigned  n_bits=max(1, log2(32/data_width))  bin_pt=0  quantization=Truncate  overflow=Wrap  use_behavioral_HDL=on  hw_selection=Fabric  pipelined=off  dbl_ovrd=off  block_type=addsub
  concat : xbsIndex_r4/Concat  num_inputs=2  dbl_ovrd=off  block_type=concat
  const : xbsIndex_r4/Constant  const=max(0, 32/data_width-1)  gui_display_data_type=Fixed-point  arith_type=Unsigned  n_bits=max(1, log2(32/data_width))  bin_pt=0  preci_type=Single  exp_width=8  frac_width=24  explicit_period=on  period=sample_rate  equ=P=C  opselect=C  inp2=PCIN>>17  opr=+  inp1=P  carry=CIN  dbl_ovrd=off  block_type=constant
      settings: block_version=11.4
  convert_addr : xbsIndex_r4/Convert  gui_display_data_type=Fixed-point  arith_type=Unsigned  n_bits=addr_width  bin_pt=0  float_type=Single  exp_bits=8  fraction_bits=24  quantization=Truncate  overflow=Wrap  en=off  latency=0  pipeline=off  dbl_ovrd=off  block_type=convert
      settings: xl_area=[0, 0, 0, 0, 0, 0, 0]
  lsw : xbsIndex_r4/Slice  nbits=max(1, log2(32/data_width))  boolean_output=off  mode=Lower Bit Location + Width  bit1=0  base1=MSB of Input  bit0=0  base0=LSB of Input  dbl_ovrd=off  block_type=slice
  manipulate : xbsIndex_r4/Constant  const=min(1, floor(32/data_width) - 1)  gui_display_data_type=Fixed-point  arith_type=Unsigned  n_bits=1  bin_pt=0  preci_type=Single  exp_width=8  frac_width=24  explicit_period=on  period=sample_rate  equ=P=C  opselect=C  inp2=PCIN>>17  opr=+  inp1=P  carry=CIN  dbl_ovrd=off  block_type=constant
      settings: block_version=11.4
  msw : xbsIndex_r4/Slice  nbits=addr_width - max(1, log2(32/data_width))  boolean_output=off  mode=Upper Bit Location + Width  bit1=0  base1=MSB of Input  bit0=0  base0=LSB of Input  dbl_ovrd=off  block_type=slice
  mux : xbsIndex_r4/Mux  inputs=2  en=off  latency=0  precision=Full  arith_type=Unsigned  n_bits=16  bin_pt=14  quantization=Truncate  overflow=Wrap  dbl_ovrd=off  block_type=mux
      settings: block_version=11.4
  out : Outport
  wires:
  convert_addr/1 -> mux/2, msw/1, lsw/1
  const/1 -> add_sub/1
  lsw/1 -> add_sub/2
  mux/1 -> out/1
  manipulate/1 -> mux/1
  concat/1 -> mux/3
  msw/1 -> concat/1
  add_sub/1 -> concat/2
  in/1 -> convert_addr/1

== system cosmic_ray_system_top/Subsystem/core_trigger_timestamps/munge_in ==
  din : Inport
  join : Subsystem  AncestorBlock=casper_library_flow_control/bus_create  mask(bus_create){inputNum=2}
      mask prompts: inputNum "Number of inputs:"
      mask init:
      | bus_create_init(gcb,...
      |     'inputNum', inputNum);
  reinterpret : xbsIndex_r4/Reinterpret  force_arith_type=on  arith_type=Unsigned  force_bin_pt=on  bin_pt=0  block_type=reinterpret
  reinterpret_out : xbsIndex_r4/Reinterpret  force_arith_type=on  arith_type=Unsigned  force_bin_pt=on  bin_pt=0  block_type=reinterpret
  split : Subsystem  AncestorBlock=casper_library_flow_control/bus_expand  mask(bus_expand){mode=divisions of arbitrary size, outputNum=1, outputWidth=[32 32], outputBinaryPt=[0 0], outputArithmeticType=[0 0], show_format=off, outputToWorkspace=off, variablePrefix=out, outputToModelAsWell=on}
      mask prompts: outputNum "Number of outputs:"; outputWidth "Output width [msb ... lsb]:"; outputBinaryPt "Output binary point position [msb ... lsb]:"; outputArithmeticType "Output arithmetic type (ufix=0, fix=1, bool=2) [msb ... lsb]:"; show_format "Print format string?"; outputToWorkspace "Output to workspace?"; variablePrefix "Variable name prefix:"; outputToModelAsWell "Output to model as well?"
      mask help:
      | Expands a 'bus' made using a bus_create or Xilinx
      | concat block.
      | The input will be divided into the specified number
      | of outputs with the specified arithmetic types.
      | Divisions are made from most significant bit.
      mask init: same as cosmic_ray_system_top/Subsystem/buffer_and_packetizer/bus_expand
      settings: AttributesFormatString=2 outputs
      mask TypeOptions mode: divisions of equal size | divisions of arbitrary size
      mask Callback mode: bus_expand_callback();
      mask Callback outputWidth: bus_expand_callback();
      mask Callback outputToWorkspace: bus_expand_callback();
  dout : Outport
  wires:
  reinterpret_out/1 -> dout/1
  din/1 -> reinterpret/1
  reinterpret/1 -> split/1(bus_in)
  join/1(bus_out) -> reinterpret_out/1
  split/2(lsb_out1) -> join/1(in1)
  split/1(msb_out2) -> join/2(in2)

== system cosmic_ray_system_top/Subsystem/core_trigger_timestamps/munge_out ==
  din : Inport
  join : Subsystem  AncestorBlock=casper_library_flow_control/bus_create  mask(bus_create){inputNum=2}
      mask prompts: inputNum "Number of inputs:"
      mask init:
      | bus_create_init(gcb,...
      |     'inputNum', inputNum);
  reinterpret : xbsIndex_r4/Reinterpret  force_arith_type=on  arith_type=Unsigned  force_bin_pt=on  bin_pt=0  block_type=reinterpret
  reinterpret_out : xbsIndex_r4/Reinterpret  force_arith_type=on  arith_type=Unsigned  force_bin_pt=on  bin_pt=0  block_type=reinterpret
  split : Subsystem  AncestorBlock=casper_library_flow_control/bus_expand  mask(bus_expand){mode=divisions of arbitrary size, outputNum=1, outputWidth=[32 32], outputBinaryPt=[0 0], outputArithmeticType=[0 0], show_format=off, outputToWorkspace=off, variablePrefix=out, outputToModelAsWell=on}
      mask prompts: outputNum "Number of outputs:"; outputWidth "Output width [msb ... lsb]:"; outputBinaryPt "Output binary point position [msb ... lsb]:"; outputArithmeticType "Output arithmetic type (ufix=0, fix=1, bool=2) [msb ... lsb]:"; show_format "Print format string?"; outputToWorkspace "Output to workspace?"; variablePrefix "Variable name prefix:"; outputToModelAsWell "Output to model as well?"
      mask help:
      | Expands a 'bus' made using a bus_create or Xilinx
      | concat block.
      | The input will be divided into the specified number
      | of outputs with the specified arithmetic types.
      | Divisions are made from most significant bit.
      mask init: same as cosmic_ray_system_top/Subsystem/buffer_and_packetizer/bus_expand
      settings: AttributesFormatString=2 outputs
      mask TypeOptions mode: divisions of equal size | divisions of arbitrary size
      mask Callback mode: bus_expand_callback();
      mask Callback outputWidth: bus_expand_callback();
      mask Callback outputToWorkspace: bus_expand_callback();
  dout : Outport
  wires:
  reinterpret_out/1 -> dout/1
  din/1 -> reinterpret/1
  reinterpret/1 -> split/1(bus_in)
  join/1(bus_out) -> reinterpret_out/1
  split/2(lsb_out1) -> join/1(in1)
  split/1(msb_out2) -> join/2(in2)

== system cosmic_ray_system_top/Subsystem/core_trigger_timestamps/sim_mem ==
  addr : Inport
  data : Inport  Port=2
  we : Inport  Port=3
  Data Type Conversion : DataTypeConversion  OutDataTypeStr=single
  Data Type Conversion1 : DataTypeConversion  OutDataTypeStr=double
  Data Type Conversion2 : DataTypeConversion  OutDataTypeStr=boolean
  sfunc : M-S-Function  FunctionName=shared_bram_sim_sfunc  Parameters=depth_bits, latency, init_vals  mask{depth_bits=addr_width, latency=csp_latency, init_vals=init_vals}
      mask prompts: depth_bits "Depth (2^?):"; latency "Latency (>=1):"; init_vals "Initial values:"
      mask Callback latency:
      | latency = str2double(get_param(gcb, 'latency'));
      | if latency < 1
      |     errordlg('Cannot have latency less than one.');
      |     set_param(gcb, 'latency', '1');
      | end
  sim_addr : xbsIndex_r4/Gateway Out  inherit_from_input=off  hdl_port=off  rows=1  columns=1  UseAsDAC=off  DACChannel='1'  interface=None  automatic_assignment=on  address_offset=hex2dec('00')  intf_name=''  intf_description=''  timing_constraint=None  locs_specified=off  LOCs={}  io_standard={}  block_type=gatewayout
  sim_data : xbsIndex_r4/Gateway Out  inherit_from_input=off  hdl_port=off  rows=1  columns=1  UseAsDAC=off  DACChannel='1'  interface=None  automatic_assignment=on  address_offset=hex2dec('00')  intf_name=''  intf_description=''  timing_constraint=None  locs_specified=off  LOCs={}  io_standard={}  block_type=gatewayout
  sim_we : xbsIndex_r4/Gateway Out  inherit_from_input=off  hdl_port=off  rows=1  columns=1  UseAsDAC=off  DACChannel='1'  interface=None  automatic_assignment=on  address_offset=hex2dec('00')  intf_name=''  intf_description=''  timing_constraint=None  locs_specified=off  LOCs={}  io_standard={}  block_type=gatewayout
  data_out : Outport
  wires:
  sfunc/1 -> data_out/1  "output"
  Data Type Conversion2/1 -> sfunc/3  "we"
  Data Type Conversion1/1 -> sfunc/2  "data_in"
  Data Type Conversion/1 -> sfunc/1  "addr"
  sim_we/1 -> Data Type Conversion2/1
  sim_data/1 -> Data Type Conversion1/1
  sim_addr/1 -> Data Type Conversion/1
  we/1 -> sim_we/1
  data/1 -> sim_data/1
  addr/1 -> sim_addr/1

== system cosmic_ray_system_top/Subsystem/counter_test_signal1/bus_create ==
  in1 : Inport
  in2 : Inport  Port=2
  in3 : Inport  Port=3
  in4 : Inport  Port=4
  in5 : Inport  Port=5
  in6 : Inport  Port=6
  in7 : Inport  Port=7
  in8 : Inport  Port=8
  in9 : Inport  Port=9
  in10 : Inport  Port=10
  in11 : Inport  Port=11
  in12 : Inport  Port=12
  in13 : Inport  Port=13
  in14 : Inport  Port=14
  in15 : Inport  Port=15
  in16 : Inport  Port=16
  concatenate : xbsIndex_r4/Concat  num_inputs=16  dbl_ovrd=off  block_type=concat
  reinterpret{1..16} (16 alike) : xbsIndex_r4/Reinterpret  force_arith_type=on  arith_type=Unsigned  force_bin_pt=on  bin_pt=0  block_type=reinterpret
      reinterpret1 settings: infoedit="Changes signal type without altering the binary representation.   You can changed the signal between signed and unsigned, and relocate the binary point.<br><br>Hardware notes: In hardware this block costs nothing.<br><br>Example:  Suppose the input is 6 bits wide, signed, with 2 fractional bits, and the output is forced to unsigned with 0 fractional bits.  Then an input of -2.0 (1110.00 in binary 2's complement) becomes an output of 56 (111000 in binary)."
      reinterpret2 settings: infoedit="Changes signal type without altering the binary representation.   You can changed the signal between signed and unsigned, and relocate the binary point.<br><br>Hardware notes: In hardware this block costs nothing.<br><br>Example:  Suppose the input is 6 bits wide, signed, with 2 fractional bits, and the output is forced to unsigned with 0 fractional bits.  Then an input of -2.0 (1110.00 in binary 2's complement) becomes an output of 56 (111000 in binary)."
  bus_out : Outport
  wires:
  concatenate/1 -> bus_out/1
  in1/1 -> reinterpret1/1
  reinterpret1/1 -> concatenate/1
  in2/1 -> reinterpret2/1
  reinterpret2/1 -> concatenate/2
  in3/1 -> reinterpret3/1
  reinterpret3/1 -> concatenate/3
  in4/1 -> reinterpret4/1
  reinterpret4/1 -> concatenate/4
  in5/1 -> reinterpret5/1
  reinterpret5/1 -> concatenate/5
  in6/1 -> reinterpret6/1
  reinterpret6/1 -> concatenate/6
  in7/1 -> reinterpret7/1
  reinterpret7/1 -> concatenate/7
  in8/1 -> reinterpret8/1
  reinterpret8/1 -> concatenate/8
  in9/1 -> reinterpret9/1
  reinterpret9/1 -> concatenate/9
  in10/1 -> reinterpret10/1
  reinterpret10/1 -> concatenate/10
  in11/1 -> reinterpret11/1
  reinterpret11/1 -> concatenate/11
  in12/1 -> reinterpret12/1
  reinterpret12/1 -> concatenate/12
  in13/1 -> reinterpret13/1
  reinterpret13/1 -> concatenate/13
  in14/1 -> reinterpret14/1
  reinterpret14/1 -> concatenate/14
  in15/1 -> reinterpret15/1
  reinterpret15/1 -> concatenate/15
  in16/1 -> reinterpret16/1
  reinterpret16/1 -> concatenate/16

== system cosmic_ray_system_top/Subsystem/counter_test_signal1/bus_create1 ==
  in1 : Inport
  in2 : Inport  Port=2
  in3 : Inport  Port=3
  in4 : Inport  Port=4
  in5 : Inport  Port=5
  in6 : Inport  Port=6
  in7 : Inport  Port=7
  in8 : Inport  Port=8
  in9 : Inport  Port=9
  in10 : Inport  Port=10
  in11 : Inport  Port=11
  in12 : Inport  Port=12
  in13 : Inport  Port=13
  in14 : Inport  Port=14
  in15 : Inport  Port=15
  in16 : Inport  Port=16
  concatenate : xbsIndex_r4/Concat  num_inputs=16  dbl_ovrd=off  block_type=concat
  reinterpret{1..16} (16 alike) : xbsIndex_r4/Reinterpret  force_arith_type=on  arith_type=Unsigned  force_bin_pt=on  bin_pt=0  block_type=reinterpret
      reinterpret1 settings: infoedit="Changes signal type without altering the binary representation.   You can changed the signal between signed and unsigned, and relocate the binary point.<br><br>Hardware notes: In hardware this block costs nothing.<br><br>Example:  Suppose the input is 6 bits wide, signed, with 2 fractional bits, and the output is forced to unsigned with 0 fractional bits.  Then an input of -2.0 (1110.00 in binary 2's complement) becomes an output of 56 (111000 in binary)."
      reinterpret2 settings: infoedit="Changes signal type without altering the binary representation.   You can changed the signal between signed and unsigned, and relocate the binary point.<br><br>Hardware notes: In hardware this block costs nothing.<br><br>Example:  Suppose the input is 6 bits wide, signed, with 2 fractional bits, and the output is forced to unsigned with 0 fractional bits.  Then an input of -2.0 (1110.00 in binary 2's complement) becomes an output of 56 (111000 in binary)."
  bus_out : Outport
  wires:
  concatenate/1 -> bus_out/1
  in1/1 -> reinterpret1/1
  reinterpret1/1 -> concatenate/1
  in2/1 -> reinterpret2/1
  reinterpret2/1 -> concatenate/2
  in3/1 -> reinterpret3/1
  reinterpret3/1 -> concatenate/3
  in4/1 -> reinterpret4/1
  reinterpret4/1 -> concatenate/4
  in5/1 -> reinterpret5/1
  reinterpret5/1 -> concatenate/5
  in6/1 -> reinterpret6/1
  reinterpret6/1 -> concatenate/6
  in7/1 -> reinterpret7/1
  reinterpret7/1 -> concatenate/7
  in8/1 -> reinterpret8/1
  reinterpret8/1 -> concatenate/8
  in9/1 -> reinterpret9/1
  reinterpret9/1 -> concatenate/9
  in10/1 -> reinterpret10/1
  reinterpret10/1 -> concatenate/10
  in11/1 -> reinterpret11/1
  reinterpret11/1 -> concatenate/11
  in12/1 -> reinterpret12/1
  reinterpret12/1 -> concatenate/12
  in13/1 -> reinterpret13/1
  reinterpret13/1 -> concatenate/13
  in14/1 -> reinterpret14/1
  reinterpret14/1 -> concatenate/14
  in15/1 -> reinterpret15/1
  reinterpret15/1 -> concatenate/15
  in16/1 -> reinterpret16/1
  reinterpret16/1 -> concatenate/16
